simulink model "rslqr_5_4_cleanup"  (R2021a)
settings: Solver=FixedStepAuto  StartTime=0.0  StopTime=10  RelTol=1e-3
values from neighbouring files (symbols this model uses):
  F = 100    [setup_env.m]    (also in setup_env_5_4.m)
undefined symbols (not defined in the file or in its folder): sslist, trimlist
libraries: dspsigops x6
settings Model: Creator=seedship  LastModifiedBy=seedship
settings SolverCC: AlgebraicLoopSolver=TrustRegion
settings DataIOCC: SaveFinalState=on  SaveOperatingPoint=on
settings OptimizationCC: ZeroExternalMemoryAtStartup=off  ZeroInternalMemoryAtStartup=off  InitFltsAndDblsToZero=on
settings DebuggingCC: SFMachineParentedDataDiag=warning
settings HardwareCC: ProdBitPerLong=64  ProdLongLongMode=on  ProdHWDeviceType=Intel->x86-64 (Linux 64)  TargetLongLongMode=on
settings RTWCC: BuildConfiguration=Faster Runs  TargetLang=C++  GenerateGPUCode=CUDA
settings GRTTargetCC: TargetLangStandard=C++03 (ISO)  CodeInterfacePackaging=C++ class

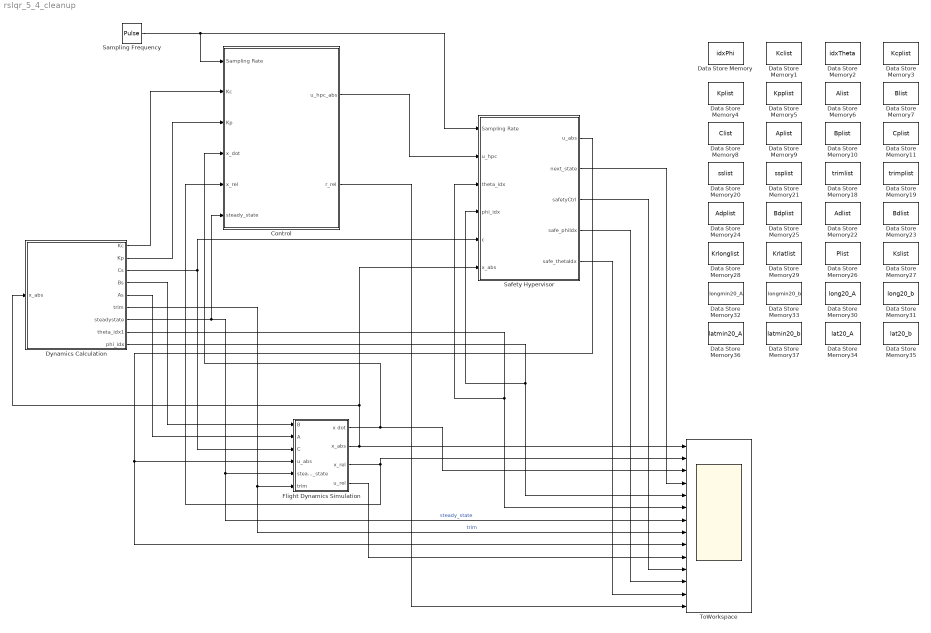
== system rslqr_5_4_cleanup ==
  Control : Subsystem
  Data Store Memory : DataStoreMemory  DataStoreName=idxPhi  ReadBeforeWriteMsg=warning  WriteAfterWriteMsg=warning  WriteAfterReadMsg=warning  InitialValue=idxPhi  VectorParams1D=off  ShowAdditionalParam=off  OutDataTypeStr=double
  Data Store Memory1 : DataStoreMemory  DataStoreName=Kclist  ReadBeforeWriteMsg=warning  WriteAfterWriteMsg=warning  WriteAfterReadMsg=warning  InitialValue=Kclist  VectorParams1D=off  ShowAdditionalParam=off  OutDataTypeStr=double
  Data Store Memory10 : DataStoreMemory  DataStoreName=Bplist  ReadBeforeWriteMsg=warning  WriteAfterWriteMsg=warning  WriteAfterReadMsg=warning  InitialValue=Bplist  VectorParams1D=off  ShowAdditionalParam=off  OutDataTypeStr=double
  Data Store Memory11 : DataStoreMemory  DataStoreName=Cplist  ReadBeforeWriteMsg=warning  WriteAfterWriteMsg=warning  WriteAfterReadMsg=warning  InitialValue=Cplist  VectorParams1D=off  ShowAdditionalParam=off  OutDataTypeStr=double
  Data Store Memory18 : DataStoreMemory  DataStoreName=trimlist  ReadBeforeWriteMsg=warning  WriteAfterWriteMsg=warning  WriteAfterReadMsg=warning  InitialValue=trimlist  VectorParams1D=off  ShowAdditionalParam=off  OutDataTypeStr=double
  Data Store Memory19 : DataStoreMemory  DataStoreName=trimplist  ReadBeforeWriteMsg=warning  WriteAfterWriteMsg=warning  WriteAfterReadMsg=warning  InitialValue=trimplist  VectorParams1D=off  ShowAdditionalParam=off  OutDataTypeStr=double
  Data Store Memory2 : DataStoreMemory  DataStoreName=idxTheta  ReadBeforeWriteMsg=warning  WriteAfterWriteMsg=warning  WriteAfterReadMsg=warning  InitialValue=idxTheta  ShowAdditionalParam=off  OutDataTypeStr=double
  Data Store Memory20 : DataStoreMemory  DataStoreName=sslist  ReadBeforeWriteMsg=warning  WriteAfterWriteMsg=warning  WriteAfterReadMsg=warning  InitialValue=sslist  VectorParams1D=off  ShowAdditionalParam=off  OutDataTypeStr=double
  Data Store Memory21 : DataStoreMemory  DataStoreName=ssplist  ReadBeforeWriteMsg=warning  WriteAfterWriteMsg=warning  WriteAfterReadMsg=warning  InitialValue=ssplist  VectorParams1D=off  ShowAdditionalParam=off  OutDataTypeStr=double
  Data Store Memory22 : DataStoreMemory  DataStoreName=Adlist  ReadBeforeWriteMsg=warning  WriteAfterWriteMsg=warning  WriteAfterReadMsg=warning  InitialValue=Adlist  VectorParams1D=off  ShowAdditionalParam=off  OutDataTypeStr=double
  Data Store Memory23 : DataStoreMemory  DataStoreName=Bdlist  ReadBeforeWriteMsg=warning  WriteAfterWriteMsg=warning  WriteAfterReadMsg=warning  InitialValue=Bdlist  VectorParams1D=off  ShowAdditionalParam=off  OutDataTypeStr=double
  Data Store Memory24 : DataStoreMemory  DataStoreName=Adplist  ReadBeforeWriteMsg=warning  WriteAfterWriteMsg=warning  WriteAfterReadMsg=warning  InitialValue=Adplist  VectorParams1D=off  ShowAdditionalParam=off  OutDataTypeStr=double
  Data Store Memory25 : DataStoreMemory  DataStoreName=Bdplist  ReadBeforeWriteMsg=warning  WriteAfterWriteMsg=warning  WriteAfterReadMsg=warning  InitialValue=Bdplist  VectorParams1D=off  ShowAdditionalParam=off  OutDataTypeStr=double
  Data Store Memory26 : DataStoreMemory  DataStoreName=Plist  ReadBeforeWriteMsg=warning  WriteAfterWriteMsg=warning  WriteAfterReadMsg=warning  InitialValue=Plist  VectorParams1D=off  ShowAdditionalParam=off  OutDataTypeStr=double
  Data Store Memory27 : DataStoreMemory  DataStoreName=Kslist  ReadBeforeWriteMsg=warning  WriteAfterWriteMsg=warning  WriteAfterReadMsg=warning  InitialValue=Kslist  VectorParams1D=off  ShowAdditionalParam=off  OutDataTypeStr=double
  Data Store Memory28 : DataStoreMemory  DataStoreName=Krlonglist  ReadBeforeWriteMsg=warning  WriteAfterWriteMsg=warning  WriteAfterReadMsg=warning  InitialValue=Krlonglist  VectorParams1D=off  ShowAdditionalParam=off  OutDataTypeStr=double
  Data Store Memory29 : DataStoreMemory  DataStoreName=Krlatlist  ReadBeforeWriteMsg=warning  WriteAfterWriteMsg=warning  WriteAfterReadMsg=warning  InitialValue=Krlatlist  VectorParams1D=off  ShowAdditionalParam=off  OutDataTypeStr=double
  Data Store Memory3 : DataStoreMemory  DataStoreName=Kcplist  ReadBeforeWriteMsg=warning  WriteAfterWriteMsg=warning  WriteAfterReadMsg=warning  InitialValue=Kcplist  ShowAdditionalParam=off  OutDataTypeStr=double
  Data Store Memory30 : DataStoreMemory  DataStoreName=long20_A  ReadBeforeWriteMsg=warning  WriteAfterWriteMsg=warning  WriteAfterReadMsg=warning  InitialValue=long20_A  VectorParams1D=off  ShowAdditionalParam=off  OutDataTypeStr=double
  Data Store Memory31 : DataStoreMemory  DataStoreName=long20_b  ReadBeforeWriteMsg=warning  WriteAfterWriteMsg=warning  WriteAfterReadMsg=warning  InitialValue=long20_b  VectorParams1D=off  ShowAdditionalParam=off  OutDataTypeStr=double
  Data Store Memory32 : DataStoreMemory  DataStoreName=longmin20_A  ReadBeforeWriteMsg=warning  WriteAfterWriteMsg=warning  WriteAfterReadMsg=warning  InitialValue=longmin20_A  VectorParams1D=off  ShowAdditionalParam=off  OutDataTypeStr=double
  Data Store Memory33 : DataStoreMemory  DataStoreName=longmin20_b  ReadBeforeWriteMsg=warning  WriteAfterWriteMsg=warning  WriteAfterReadMsg=warning  InitialValue=longmin20_A  VectorParams1D=off  ShowAdditionalParam=off  OutDataTypeStr=double
  Data Store Memory34 : DataStoreMemory  DataStoreName=lat20_A  ReadBeforeWriteMsg=warning  WriteAfterWriteMsg=warning  WriteAfterReadMsg=warning  InitialValue=lat20_A  VectorParams1D=off  ShowAdditionalParam=off  OutDataTypeStr=double
  Data Store Memory35 : DataStoreMemory  DataStoreName=lat20_b  ReadBeforeWriteMsg=warning  WriteAfterWriteMsg=warning  WriteAfterReadMsg=warning  InitialValue=lat20_b  VectorParams1D=off  ShowAdditionalParam=off  OutDataTypeStr=double
  Data Store Memory36 : DataStoreMemory  DataStoreName=latmin20_A  ReadBeforeWriteMsg=warning  WriteAfterWriteMsg=warning  WriteAfterReadMsg=warning  InitialValue=latmin20_A  VectorParams1D=off  ShowAdditionalParam=off  OutDataTypeStr=double
  Data Store Memory37 : DataStoreMemory  DataStoreName=latmin20_b  ReadBeforeWriteMsg=warning  WriteAfterWriteMsg=warning  WriteAfterReadMsg=warning  InitialValue=latmin20_b  VectorParams1D=off  ShowAdditionalParam=off  OutDataTypeStr=double
  Data Store Memory4 : DataStoreMemory  DataStoreName=Kplist  ReadBeforeWriteMsg=warning  WriteAfterWriteMsg=warning  WriteAfterReadMsg=warning  InitialValue=Kplist  ShowAdditionalParam=off  OutDataTypeStr=double
  Data Store Memory5 : DataStoreMemory  DataStoreName=Kpplist  ReadBeforeWriteMsg=warning  WriteAfterWriteMsg=warning  WriteAfterReadMsg=warning  InitialValue=Kpplist  ShowAdditionalParam=off  OutDataTypeStr=double
  Data Store Memory6 : DataStoreMemory  DataStoreName=Alist  ReadBeforeWriteMsg=warning  WriteAfterWriteMsg=warning  WriteAfterReadMsg=warning  InitialValue=Alist  VectorParams1D=off  ShowAdditionalParam=off  OutDataTypeStr=double
  Data Store Memory7 : DataStoreMemory  DataStoreName=Blist  ReadBeforeWriteMsg=warning  WriteAfterWriteMsg=warning  WriteAfterReadMsg=warning  InitialValue=Blist  VectorParams1D=off  ShowAdditionalParam=off  OutDataTypeStr=double
  Data Store Memory8 : DataStoreMemory  DataStoreName=Clist  ReadBeforeWriteMsg=warning  WriteAfterWriteMsg=warning  WriteAfterReadMsg=warning  InitialValue=Clist  VectorParams1D=off  ShowAdditionalParam=off  OutDataTypeStr=double
  Data Store Memory9 : DataStoreMemory  DataStoreName=Aplist  ReadBeforeWriteMsg=warning  WriteAfterWriteMsg=warning  WriteAfterReadMsg=warning  InitialValue=Aplist  VectorParams1D=off  ShowAdditionalParam=off  OutDataTypeStr=double
  Dynamics Calculation : Subsystem
  Flight Dynamics Simulation : Subsystem
  Safety Hypervisor : Subsystem
  Sampling Frequency : DiscretePulseGenerator  PulseType=Time based  Period=1/F  PulseWidth=50
  ToWorkspace : Scope  NumInputPorts=14
  wires:
  Sampling Frequency/1 -> Control/1(Sampling Rate), Safety Hypervisor/1(Sampling Rate)
  Dynamics Calculation/6(trim) -> ToWorkspace/8, Flight Dynamics Simulation/6(trim)  "trim"
  Dynamics Calculation/7(steadystate) -> Flight Dynamics Simulation/5(steady_state), ToWorkspace/7, Control/6(steady_state)  "steady_state"
  Flight Dynamics Simulation/1(x dot) -> Control/4(x_dot), ToWorkspace/3
  Flight Dynamics Simulation/3(x_rel) -> Control/5(x_rel), ToWorkspace/2
  Dynamics Calculation/4(Bs) -> Flight Dynamics Simulation/1(B)
  Dynamics Calculation/5(As) -> Flight Dynamics Simulation/2(A)
  Flight Dynamics Simulation/4(u_rel) -> ToWorkspace/10
  Dynamics Calculation/1(Kc) -> Control/2(Kc)
  Dynamics Calculation/2(Kp) -> Control/3(Kp)
  Control/2(r_rel) -> ToWorkspace/14
  Flight Dynamics Simulation/2(x_abs) -> Safety Hypervisor/6(x_abs), Dynamics Calculation/1(x_abs), ToWorkspace/1
  Dynamics Calculation/9(phi_idx) -> Safety Hypervisor/4(phi_idx), ToWorkspace/5
  Dynamics Calculation/8(theta_idx1) -> ToWorkspace/6, Safety Hypervisor/3(theta_idx)
  Dynamics Calculation/3(Cs) -> Flight Dynamics Simulation/3(C), Safety Hypervisor/5(c)
  Safety Hypervisor/1(u_abs) -> ToWorkspace/9, Flight Dynamics Simulation/4(u_abs)
  Control/1(u_hpc_abs) -> Safety Hypervisor/2(u_hpc)
  Safety Hypervisor/2(next_state) -> ToWorkspace/4
  Safety Hypervisor/3(safetyCtrl) -> ToWorkspace/11
  Safety Hypervisor/4(safe_phiIdx) -> ToWorkspace/12
  Safety Hypervisor/5(safe_thetaIdx) -> ToWorkspace/13

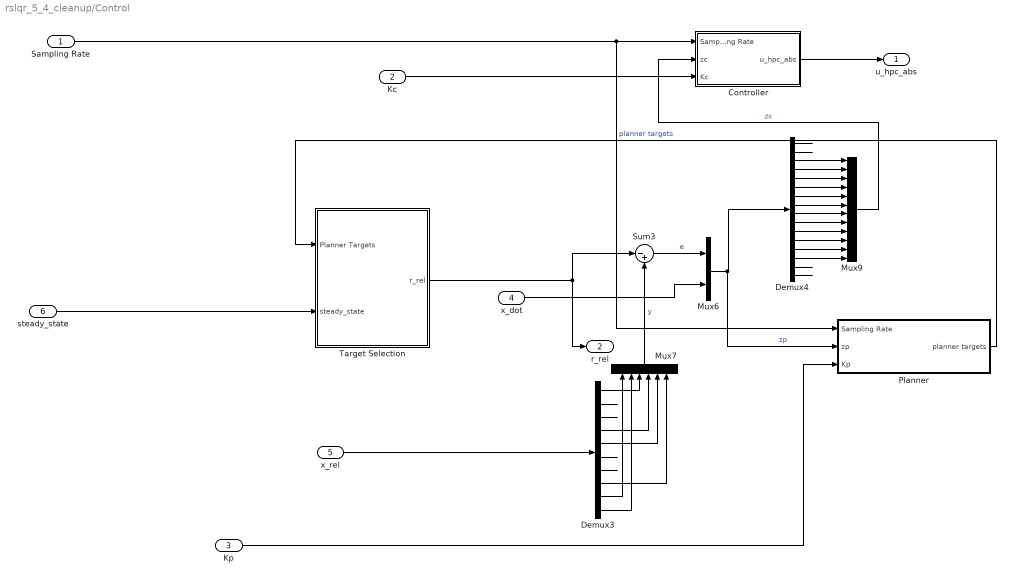
== system rslqr_5_4_cleanup/Control ==
  Sampling Rate : Inport
  Kc : Inport  Port=2
  Kp : Inport  Port=3
  x_dot : Inport  Port=4
  x_rel : Inport  Port=5
  steady_state : Inport  Port=6
  Controller : Subsystem
  Demux3 : Demux  Outputs=10
  Demux4 : Demux  Outputs=16
  Mux6 : Mux  Inputs=2
  Mux7 : Mux  Inputs=6
  Mux9 : Mux  Inputs=12
  Planner : Subsystem
  Sum3 : Sum  Inputs=|-+
  Target Selection : Subsystem
  u_hpc_abs : Outport
  r_rel : Outport  Port=2
  wires:
  Kc/1 -> Controller/3(Kc)
  Demux3/6 -> ?
  Demux4/3 -> Mux9/1
  Mux6/1 -> Planner/2(zp), Demux4/1  "zp"
  Kp/1 -> Planner/3(Kp)
  Demux4/8 -> Mux9/6
  Demux4/11 -> Mux9/9
  Demux3/7 -> ?
  Planner/1(planner targets) -> Target Selection/1(Planner Targets)  "planner targets"
  Demux4/6 -> Mux9/4
  Demux4/10 -> Mux9/8
  x_dot/1 -> Mux6/2
  Demux4/1 -> ?
  Demux3/8 -> Mux7/6
  Demux4/14 -> Mux9/12
  Sampling Rate/1 -> Planner/1(Sampling Rate), Controller/1(Sampling Rate)
  Target Selection/1(r_rel) -> r_rel/1, Sum3/1
  Demux4/16 -> ?
  Demux4/13 -> Mux9/11
  Demux4/15 -> ?
  Demux4/4 -> Mux9/2
  x_rel/1 -> Demux3/1
  steady_state/1 -> Target Selection/2(steady_state)
  Demux4/2 -> ?
  Sum3/1 -> Mux6/1  "e"
  Demux3/10 -> Mux7/2
  Mux9/1 -> Controller/2(zc)  "zc"
  Demux3/3 -> ?
  Demux4/12 -> Mux9/10
  Demux3/2 -> ?
  Demux3/4 -> Mux7/4
  Controller/1(u_hpc_abs) -> u_hpc_abs/1
  Demux4/9 -> Mux9/7
  Mux7/1 -> Sum3/2  "y"
  Demux3/9 -> Mux7/1
  Demux4/7 -> Mux9/5
  Demux3/5 -> Mux7/5
  Demux4/5 -> Mux9/3
  Demux3/1 -> Mux7/3

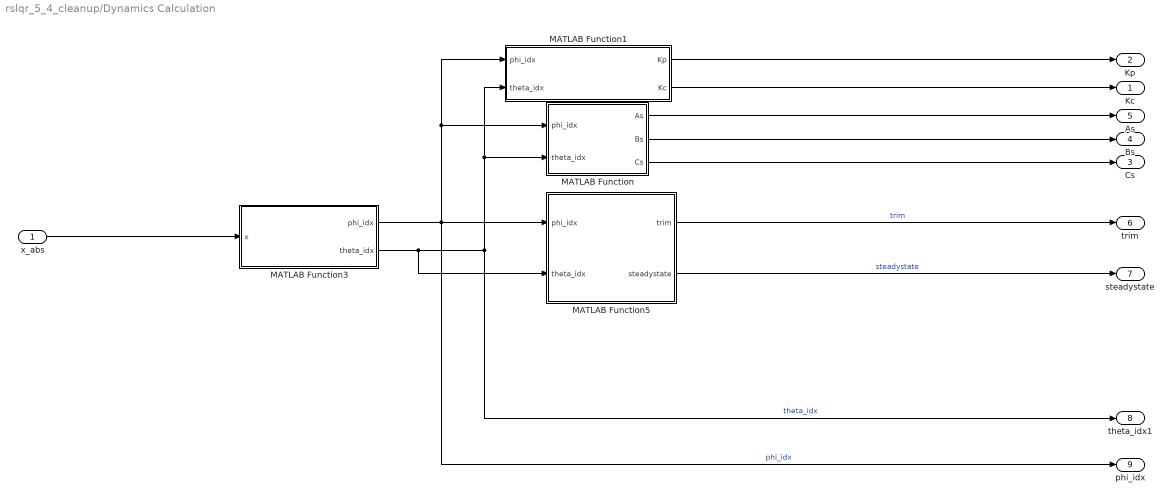
== system rslqr_5_4_cleanup/Dynamics Calculation ==
  x_abs : Inport
  MATLAB Function : MATLAB Function  TreatAsAtomicUnit=on
  MATLAB Function1 : MATLAB Function  TreatAsAtomicUnit=on
  MATLAB Function3 : MATLAB Function  TreatAsAtomicUnit=on
  MATLAB Function5 : MATLAB Function  TreatAsAtomicUnit=on
  Kc : Outport
  Kp : Outport  Port=2
  Cs : Outport  Port=3
  Bs : Outport  Port=4
  As : Outport  Port=5
  trim : Outport  Port=6
  steadystate : Outport  Port=7
  theta_idx1 : Outport  Port=8
  phi_idx : Outport  Port=9
  wires:
  x_abs/1 -> MATLAB Function3/1(x)
  MATLAB Function/3(Cs) -> Cs/1
  MATLAB Function3/1(phi_idx) -> phi_idx/1, MATLAB Function5/1(phi_idx), MATLAB Function1/1(phi_idx), MATLAB Function/1(phi_idx)  "phi_idx"
  MATLAB Function5/1(trim) -> trim/1  "trim"
  MATLAB Function/1(As) -> As/1
  MATLAB Function1/2(Kc) -> Kc/1
  MATLAB Function5/2(steadystate) -> steadystate/1  "steadystate"
  MATLAB Function1/1(Kp) -> Kp/1
  MATLAB Function3/2(theta_idx) -> MATLAB Function5/2(theta_idx), MATLAB Function1/2(theta_idx), MATLAB Function/2(theta_idx), theta_idx1/1  "theta_idx"
  MATLAB Function/2(Bs) -> Bs/1

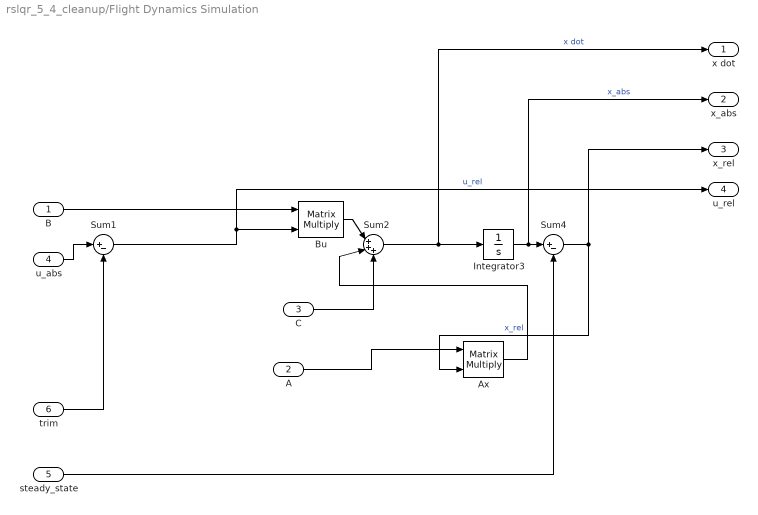
== system rslqr_5_4_cleanup/Flight Dynamics Simulation ==
  B : Inport
  A : Inport  Port=2
  C : Inport  Port=3
  u_abs : Inport  Port=4
  steady_state : Inport  Port=5
  trim : Inport  Port=6
  Ax : Product  Multiplication=Matrix(*)
  Bu : Product  Multiplication=Matrix(*)
  Integrator3 : Integrator  InitialCondition=sslist(:,3)
  Sum1 : Sum  Inputs=|+-
  Sum2 : Sum  Inputs=|+++
  Sum4 : Sum  Inputs=|+-
  x dot : Outport
  x_abs : Outport  Port=2
  x_rel : Outport  Port=3
  u_rel : Outport  Port=4
  wires:
  A/1 -> Ax/1
  Sum4/1 -> x_rel/1, Ax/2  "x_rel"
  Ax/1 -> Sum2/2
  Bu/1 -> Sum2/1
  B/1 -> Bu/1
  u_abs/1 -> Sum1/1
  trim/1 -> Sum1/2
  Sum2/1 -> Integrator3/1, x dot/1  "x dot"
  C/1 -> Sum2/3
  Sum1/1 -> Bu/2, u_rel/1  "u_rel"
  Integrator3/1 -> x_abs/1, Sum4/1  "x_abs"
  steady_state/1 -> Sum4/2

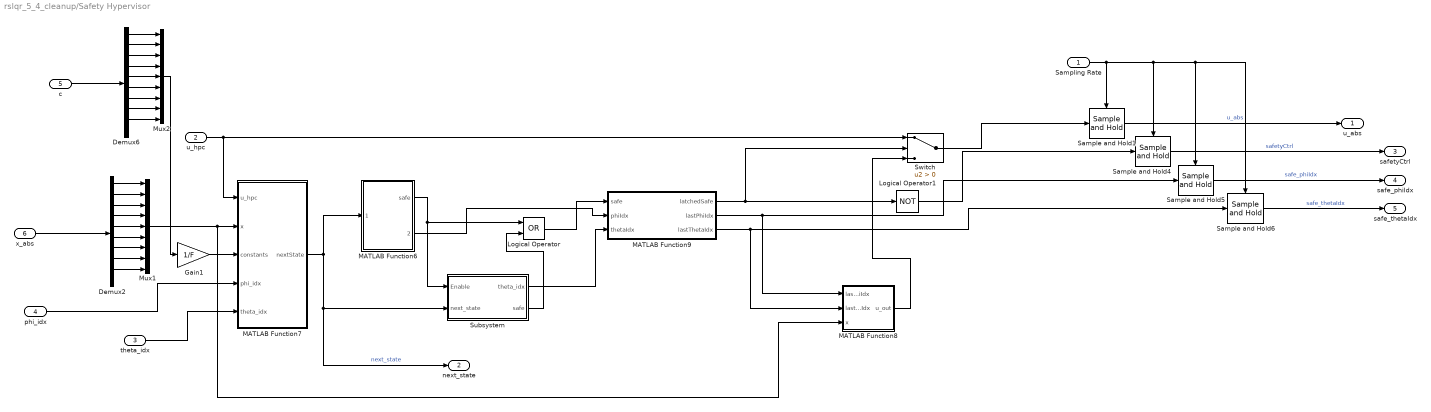
== system rslqr_5_4_cleanup/Safety Hypervisor ==
  Sampling Rate : Inport
  u_hpc : Inport  Port=2
  theta_idx : Inport  Port=3
  phi_idx : Inport  Port=4
  c : Inport  Port=5
  x_abs : Inport  Port=6
  Demux2 : Demux  Outputs=10
  Demux6 : Demux  Outputs=10
  Gain1 : Gain  Gain=1/F
  Logical Operator : Logic  Operator=OR  AllPortsSameDT=off  OutDataTypeStr=boolean
  Logical Operator1 : Logic  Operator=NOT  Inputs=1  AllPortsSameDT=off  OutDataTypeStr=boolean
  MATLAB Function6 : MATLAB Function  TreatAsAtomicUnit=on
  MATLAB Function7 : MATLAB Function  TreatAsAtomicUnit=on
  MATLAB Function8 : MATLAB Function  TreatAsAtomicUnit=on
  MATLAB Function9 : MATLAB Function  TreatAsAtomicUnit=on
  Mux1 : Mux  Inputs=9
  Mux2 : Mux  Inputs=9
  Sample and Hold{1,4..6} (4 alike) : dspsigops/Sample and Hold  trig=Rising edge  initCond=0  latchinput=off
  Subsystem : Subsystem
  Switch : Switch  Criteria=u2 > Threshold
  u_abs : Outport
  next_state : Outport  Port=2
  safetyCtrl : Outport  Port=3
  safe_phiIdx : Outport  Port=4
  safe_thetaIdx : Outport  Port=5
  wires:
  Demux6/7 -> Mux2/7
  Demux2/4 -> Mux1/4
  Demux6/6 -> Mux2/6
  Logical Operator1/1 -> Sample and Hold4/1
  Sample and Hold5/1 -> safe_phiIdx/1  "safe_phiIdx"
  Demux2/8 -> Mux1/8
  Sample and Hold6/1 -> safe_thetaIdx/1  "safe_thetaIdx"
  Demux6/9 -> Mux2/9
  phi_idx/1 -> MATLAB Function7/4(phi_idx)
  Subsystem/2(safe) -> Logical Operator/2
  MATLAB Function9/2(lastPhiIdx) -> Sample and Hold5/1, MATLAB Function8/1(lastPhiIdx)
  MATLAB Function9/1(latchedSafe) -> Logical Operator1/1, Switch/2
  MATLAB Function6/1(safe) -> Subsystem/1(Enable), Logical Operator/1
  MATLAB Function7/1(nextState) -> next_state/1, Subsystem/2(next_state), MATLAB Function6/1(nextState)  "next_state"
  Demux6/2 -> Mux2/2
  Demux2/5 -> Mux1/5
  Logical Operator/1 -> MATLAB Function9/1(safe)
  c/1 -> Demux6/1
  Demux2/3 -> Mux1/3
  Switch/1 -> Sample and Hold1/1
  Sample and Hold4/1 -> safetyCtrl/1  "safetyCtrl"
  x_abs/1 -> Demux2/1
  Subsystem/1(theta_idx) -> MATLAB Function9/3(thetaIdx)
  Demux6/1 -> Mux2/1
  Demux6/8 -> Mux2/8
  Demux2/9 -> Mux1/9
  Demux2/6 -> Mux1/6
  Demux2/2 -> Mux1/2
  Demux6/3 -> Mux2/3
  Demux2/1 -> Mux1/1
  Demux6/5 -> Mux2/5
  Demux2/7 -> Mux1/7
  Sample and Hold1/1 -> u_abs/1  "u_abs"
  Gain1/1 -> MATLAB Function7/3(constants)
  theta_idx/1 -> MATLAB Function7/5(theta_idx)
  MATLAB Function9/3(lastThetaIdx) -> Sample and Hold6/1, MATLAB Function8/2(lastThetaIdx)
  u_hpc/1 -> MATLAB Function7/1(u_hpc), Switch/1
  Mux2/1 -> Gain1/1
  MATLAB Function8/1(u_out) -> Switch/3
  Sampling Rate/1 -> Sample and Hold1/Trigger, Sample and Hold4/Trigger, Sample and Hold5/Trigger, Sample and Hold6/Trigger
  Demux6/4 -> Mux2/4
  MATLAB Function6/2(safePhiIdx) -> MATLAB Function9/2(phiIdx)
  Mux1/1 -> MATLAB Function8/3(x), MATLAB Function7/2(x)

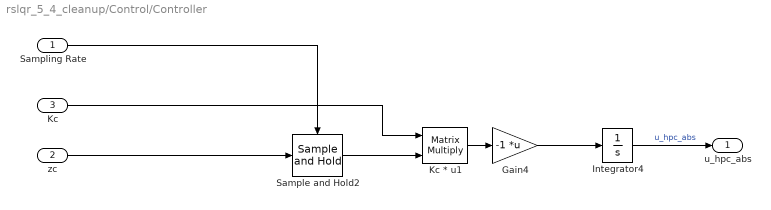
== system rslqr_5_4_cleanup/Control/Controller ==
  Sampling Rate : Inport
  zc : Inport  Port=2
  Kc : Inport  Port=3
  Gain4 : Gain  Gain=-1  Multiplication=Matrix(K*u)
  Integrator4 : Integrator  InitialCondition=trimlist(:,3)  LimitOutput=on  UpperSaturationLimit=[1 1 1 1]  LowerSaturationLimit=[ -1 -1 -1 -1]
  Kc * u1 : Product  Multiplication=Matrix(*)
  Sample and Hold2 : dspsigops/Sample and Hold  trig=Rising edge  initCond=0  latchinput=off
  u_hpc_abs : Outport
  wires:
  Sampling Rate/1 -> Sample and Hold2/Trigger
  Sample and Hold2/1 -> Kc * u1/2
  Gain4/1 -> Integrator4/1
  zc/1 -> Sample and Hold2/1
  Kc/1 -> Kc * u1/1
  Kc * u1/1 -> Gain4/1
  Integrator4/1 -> u_hpc_abs/1  "u_hpc_abs"

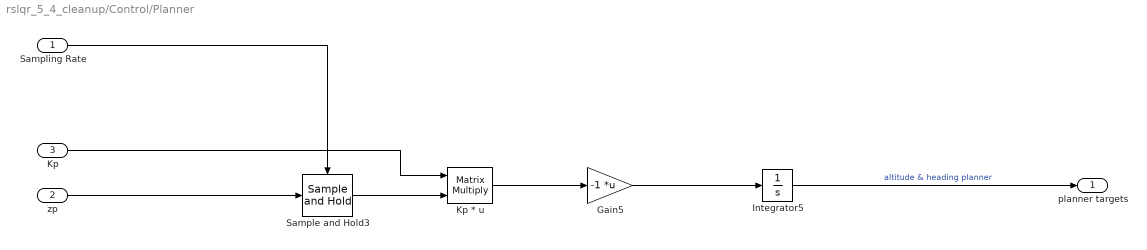
== system rslqr_5_4_cleanup/Control/Planner ==
  Sampling Rate : Inport
  zp : Inport  Port=2
  Kp : Inport  Port=3
  Gain5 : Gain  Gain=-1  Multiplication=Matrix(K*u)
  Integrator5 : Integrator  LimitOutput=on  UpperSaturationLimit=[deg2rad(50); deg2rad(70)]  LowerSaturationLimit=[-deg2rad(50); -deg2rad(70)]
  Kp * u : Product  Multiplication=Matrix(*)
  Sample and Hold3 : dspsigops/Sample and Hold  trig=Rising edge  initCond=0  latchinput=off
  planner targets : Outport
  wires:
  zp/1 -> Sample and Hold3/1
  Kp/1 -> Kp * u/1
  Kp * u/1 -> Gain5/1
  Gain5/1 -> Integrator5/1
  Integrator5/1 -> planner targets/1  "altitude & heading planner"
  Sample and Hold3/1 -> Kp * u/2
  Sampling Rate/1 -> Sample and Hold3/Trigger

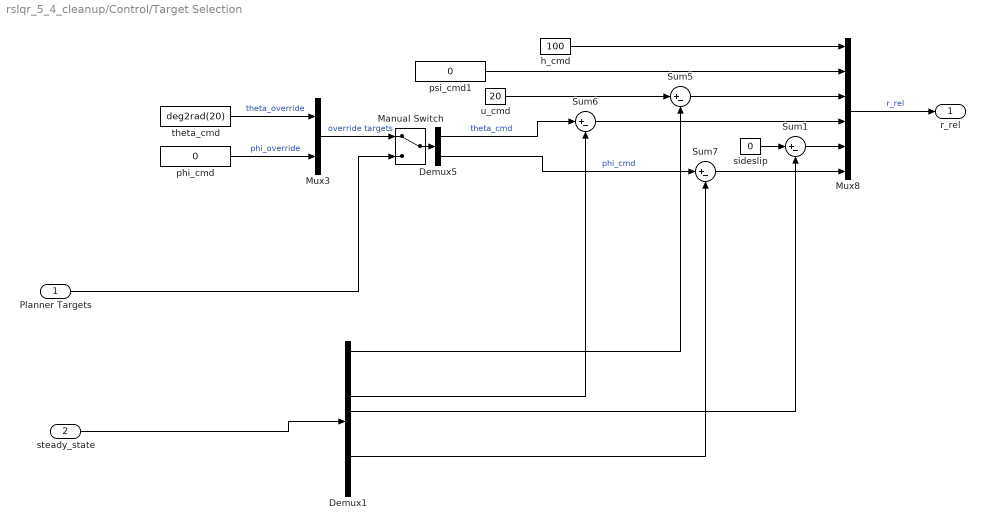
== system rslqr_5_4_cleanup/Control/Target Selection ==
  Planner Targets : Inport
  steady_state : Inport  Port=2
  Demux1 : Demux  Outputs=10
  Demux5 : Demux  Outputs=2
  Manual Switch : ManualSwitch
  Mux3 : Mux  Inputs=2
  Mux8 : Mux  Inputs=6
  Sum{1,5..7} (4 alike) : Sum  Inputs=|+-
  h_cmd : Constant  Value=100
  phi_cmd : Constant  Value=0
  psi_cmd1 : Constant  Value=0
  sideslip : Constant  Value=0
  theta_cmd : Constant  Value=deg2rad(20)
  u_cmd : Constant  Value=20
  r_rel : Outport
  wires:
  steady_state/1 -> Demux1/1
  Manual Switch/1 -> Demux5/1
  psi_cmd1/1 -> Mux8/2
  Planner Targets/1 -> Manual Switch/2
  theta_cmd/1 -> Mux3/1  "theta_override"
  Sum5/1 -> Mux8/3
  Mux8/1 -> r_rel/1  "r_rel"
  Demux1/4 -> Sum6/2
  Demux5/2 -> Sum7/1  "phi_cmd"
  Demux5/1 -> Sum6/1  "theta_cmd"
  Demux1/8 -> Sum7/2
  u_cmd/1 -> Sum5/1
  Sum7/1 -> Mux8/6
  phi_cmd/1 -> Mux3/2  "phi_override"
  Demux1/1 -> Sum5/2
  Sum6/1 -> Mux8/4
  h_cmd/1 -> Mux8/1
  Mux3/1 -> Manual Switch/1  "override targets"
  sideslip/1 -> Sum1/1
  Sum1/1 -> Mux8/5
  Demux1/5 -> Sum1/2

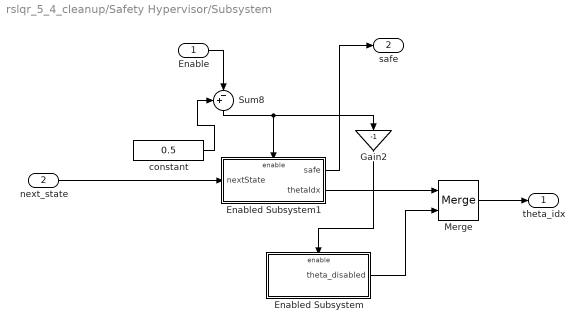
== system rslqr_5_4_cleanup/Safety Hypervisor/Subsystem ==
  Enable : Inport
  next_state : Inport  Port=2
  Enabled Subsystem : Subsystem  TreatAsAtomicUnit=on
  Enabled Subsystem1 : Subsystem  TreatAsAtomicUnit=on
  Gain2 : Gain  Gain=-1
  Merge : Merge
  Sum8 : Sum  Inputs=+-|
  constant : Constant  Value=0.5
  theta_idx : Outport
  safe : Outport  Port=2
  wires:
  Enable/1 -> Sum8/2
  Sum8/1 -> Gain2/1, Enabled Subsystem1/Enable
  Enabled Subsystem1/1(safe) -> safe/1
  Enabled Subsystem1/2(thetaIdx) -> Merge/1
  Enabled Subsystem/1(theta_disabled) -> Merge/2
  Gain2/1 -> Enabled Subsystem/Enable
  next_state/1 -> Enabled Subsystem1/1(nextState)
  Merge/1 -> theta_idx/1
  constant/1 -> Sum8/1

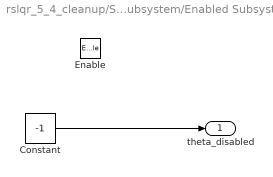
== system rslqr_5_4_cleanup/Safety Hypervisor/Subsystem/Enabled Subsystem ==
  Enable : EnablePort
  Constant : Constant  Value=-1
  theta_disabled : Outport
  wires:
  Constant/1 -> theta_disabled/1

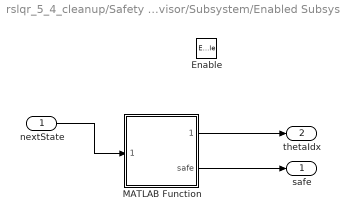
== system rslqr_5_4_cleanup/Safety Hypervisor/Subsystem/Enabled Subsystem1 ==
  nextState : Inport
  Enable : EnablePort
  MATLAB Function : MATLAB Function  TreatAsAtomicUnit=on
  safe : Outport  InitialOutput=0  VectorParamsAs1DForOutWhenUnconnected=off
  thetaIdx : Outport  Port=2  InitialOutput=0  VectorParamsAs1DForOutWhenUnconnected=off
  wires:
  nextState/1 -> MATLAB Function/1(nextState)
  MATLAB Function/1(safeThetaIdx) -> thetaIdx/1
  MATLAB Function/2(safe) -> safe/1

== matlab function rslqr_5_4_cleanup/Safety Hypervisor/Subsystem/Enabled Subsystem1/MATLAB Function ==
  data: nextState input; safeThetaIdx output; lat20_A data_store_memory; lat20_b data_store_memory; latmin20_A data_store_memory; latmin20_b data_store_memory; long20_A data_store_memory; long20_b data_store_memory; longmin20_A data_store_memory; longmin20_b data_store_memory; safe output; ssplist data_store_memory
function [safeThetaIdx,safe] = recoverableRegionPitch(nextState)
    global ssplist long20_A long20_b lat20_A lat20_b longmin20_A longmin20_b latmin20_A latmin20_b
    safe = 0;
    safeThetaIdx = -1;
    %% Test pitch reachability +20 deg
    x_hat = nextState - ssplist(1:9, 3);
    x_hat_long = x_hat([1:4,9]);
    x_hat_lat = x_hat(5:8);
    if polyContains(long20_A, long20_b, x_hat_long) && polyContains(lat20_A, lat20_b, x_hat_lat)
       safe = 1;
       safeThetaIdx = 3;
    end
    
    %% Test pitch reachability -20 deg
    x_hat = nextState - ssplist(1:9, 1);
    x_hat_long = x_hat([1:4,9]);
    x_hat_lat = x_hat(5:8);
    if polyContains(longmin20_A, longmin20_b, x_hat_long) && polyContains(latmin20_A, latmin20_b, x_hat_lat)
       safe = 1;
       safeThetaIdx = 1;
    end
end

== matlab function rslqr_5_4_cleanup/Safety Hypervisor/MATLAB Function8 ==
  settings: updateMethod=DISCRETE
  data: lastPhiIdx input; u_out output; trimplist data_store_memory; trimlist data_store_memory; ssplist data_store_memory; sslist data_store_memory; lastThetaIdx input; Kslist data_store_memory; Krlonglist data_store_memory; Krlatlist data_store_memory; x input
function u_out = safetyCtrl(lastPhiIdx, lastThetaIdx, x)
    global Kslist sslist trimlist Krlonglist ssplist Krlatlist trimplist
    if lastPhiIdx ~= -1
        u_out = bound(-Kslist(:,:,lastPhiIdx) * (x - sslist(1:9, lastPhiIdx)), -1, 1) + trimlist(:, lastPhiIdx);
    elseif lastThetaIdx == 1 || lastThetaIdx == 3
        xlong = x([1:4,9]);
        xlat = x(5:8);
        u_out = [-Krlonglist(:,:,lastThetaIdx) * (xlong - ssplist([1:4,9], lastThetaIdx));
                 -Krlatlist(:,:,lastThetaIdx) * (xlat - ssplist(5:8, lastThetaIdx))];
        u_out = bound(u_out, -1, 1) + trimplist(:, lastThetaIdx);
    else
        error('Error! lastThetaIdx: %i\n', lastThetaIdx)
    end
end

function y = bound(x,bl,bu)
  % return bounded value clipped between bl and bu
  y=min(max(x,bl),bu);
end

== matlab function rslqr_5_4_cleanup/Safety Hypervisor/MATLAB Function9 ==
  data: safe input; latchedSafe output; phiIdx input; thetaIdx input; lastPhiIdx output; lastThetaIdx output
function [latchedSafe, lastPhiIdx, lastThetaIdx] = isSafe(safe, phiIdx, thetaIdx)
    persistent latchedSafe_p lastPhiIdx_p lastThetaIdx_p

    if isempty(latchedSafe_p)
        latchedSafe_p = true;
    end
    if isempty(lastPhiIdx_p)
        lastPhiIdx_p = 3;
    end
    if isempty(lastThetaIdx_p)
        lastThetaIdx_p = -1;
    end
    
    latchedSafe_p = latchedSafe_p & safe;
    if safe
        lastPhiIdx_p = phiIdx;
        lastThetaIdx_p = thetaIdx;
    end
    
    latchedSafe = latchedSafe_p;
    lastPhiIdx = lastPhiIdx_p;
    lastThetaIdx = lastThetaIdx_p;
end

== matlab function rslqr_5_4_cleanup/Dynamics Calculation/MATLAB Function1 ==
  settings: updateMethod=DISCRETE
  data: phi_idx input; Kclist data_store_memory; Kplist data_store_memory; Kcplist data_store_memory; Kpplist data_store_memory; Kp output size=[2 16]; Kc output size=[4 12]; theta_idx input
function [Kp,Kc] = calculateRSLQRGains(phi_idx, theta_idx)
    % Nearest A, B
    global Kclist Kplist Kcplist Kpplist
    
    
    if theta_idx ~= 2
        Kc = Kcplist(:,:, theta_idx);
        Kp = Kpplist(:,:, theta_idx);
        return
    end
    
    Kc = Kclist(:,:, phi_idx);
    Kp = Kplist(:,:, phi_idx);
end

== matlab function rslqr_5_4_cleanup/Dynamics Calculation/MATLAB Function ==
  settings: updateMethod=DISCRETE
  data: phi_idx input; Alist data_store_memory; Aplist data_store_memory; Blist data_store_memory; Bplist data_store_memory; Clist data_store_memory; Cplist data_store_memory; As output size=[10 10]; Bs output size=[10 4]; Cs output size=10; theta_idx input
function [As,Bs, Cs] = calculateDynamics(phi_idx, theta_idx)
    % Nearest A, B
    global Alist Blist Clist Aplist Bplist Cplist;
    
    if theta_idx ~= 2
        As = Aplist(:,:, theta_idx);
        Bs = Bplist(:,:, theta_idx);
        Cs = Cplist(:, theta_idx);
        return
    end
    
    As = Alist(:,:, phi_idx);
    Bs = Blist(:,:, phi_idx);
    Cs = Clist(:, phi_idx);
end

== matlab function rslqr_5_4_cleanup/Dynamics Calculation/MATLAB Function3 ==
  settings: updateMethod=DISCRETE
  data: x input; idxPhi data_store_memory; idxTheta data_store_memory; phi_idx output size=1; theta_idx output size=1
function [phi_idx, theta_idx]= calculateIdx(x)
    % Nearest A, B
    global idxPhi idxTheta
    [~, phi_idx] = min(abs(x(8) - idxPhi));
    [~, theta_idx] = min(abs(x(4) - idxTheta));
end

== matlab function rslqr_5_4_cleanup/Dynamics Calculation/MATLAB Function5 ==
  settings: updateMethod=DISCRETE
  data: phi_idx input; trim output size=4; steadystate output size=10; theta_idx input; trimlist data_store_memory; trimplist data_store_memory; sslist data_store_memory; ssplist data_store_memory
function [trim, steadystate] = calculateTrimSteadyState(phi_idx, theta_idx)
    % Nearest A, B
    global trimlist trimplist sslist ssplist;
    
    if theta_idx ~= 2
        trim = trimplist(:, theta_idx);
        steadystate = ssplist(:, theta_idx);
        return
    end
    
    trim = trimlist(:, phi_idx);
    steadystate = sslist(:, phi_idx);
end

== matlab function rslqr_5_4_cleanup/Safety Hypervisor/MATLAB Function6 ==
  data: nextState input; safe output; safePhiIdx output; sslist data_store_memory; Plist data_store_memory
function [safe, safePhiIdx] = recoverableRegionSimplex(nextState)

    global sslist Plist

    safe = 0;
    safePhiIdx = -1;
    for idx = [3,2,4,1,5]
        x_hat = nextState - sslist(1:9, idx);
        if x_hat' * Plist(:,:,idx) * x_hat < 1
            safe = 1;
            safePhiIdx = idx;
            return
        end
    end

== matlab function rslqr_5_4_cleanup/Safety Hypervisor/MATLAB Function7 ==
  settings: updateMethod=DISCRETE
  data: u_hpc input; nextState output; x input; constants input; phi_idx input; theta_idx input; Adplist data_store_memory; Adlist data_store_memory; Bdlist data_store_memory; Bdplist data_store_memory; sslist data_store_memory; ssplist data_store_memory; trimlist data_store_memory; trimplist data_store_memory
function nextState = calculateNextState(u_hpc, x, constants, phi_idx, theta_idx)

    global Adlist Adplist Bdlist Bdplist sslist ssplist trimlist trimplist

    %% Calculate next state
    if theta_idx ~= 2
        % Handle pitch reachability
        nextState = Adplist(:,:,theta_idx) * (x - ssplist(1:9, theta_idx)) + Bdplist(:,:,theta_idx) * (u_hpc - trimplist(:, theta_idx)) + constants + ssplist(1:9, theta_idx);
    else
        nextState = Adlist(:,:,phi_idx) * (x - sslist(1:9, phi_idx)) + Bdlist(:,:,phi_idx) * (u_hpc - trimlist(:, phi_idx)) + constants + sslist(1:9, phi_idx);
    end
end
